simulink model "pyrolysis_adaptive_pid"  (R2024a)
settings: Solver=ode4  StartTime=0.0  StopTime=1800  FixedStep=0.05  RelTol=1e-3
InitFcn:
  | if ~exist('setpoint_ws','var'), setpoint_ws = 300; end
  | if ~exist('gs_enable_ws','var'), gs_enable_ws = 1; end
  | if ~exist('lambda_p_ws','var'), lambda_p_ws = 0.01; end
  | if ~exist('lambda_i_ws','var'), lambda_i_ws = 0.0001; end
  | if ~exist('lambda_d_ws','var'), lambda_d_ws = 0.003; end
  | if ~exist('noise_variance_ws','var'), noise_variance_ws = 2.25; end
undefined symbols (not defined in the file or in its folder): gs_enable_ws, lambda_d_ws, lambda_i_ws, lambda_p_ws, setpoint_ws
libraries: simulink x1
settings Model: Creator=indie  LastModifiedBy=indie

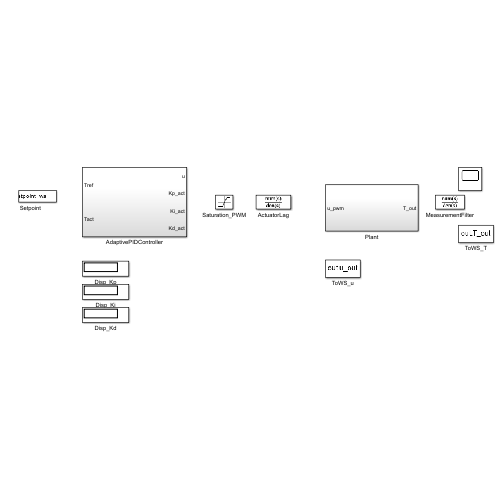
[thumbnail: Simulink's stored preview of the top-level diagram]
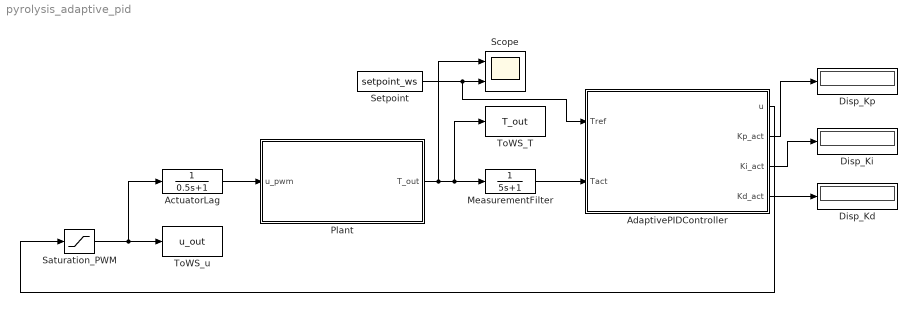
== system pyrolysis_adaptive_pid ==
  ActuatorLag : TransferFcn  Denominator=[0.5 1]
  AdaptivePIDController : Subsystem
  Disp_Kd : Display
  Disp_Ki : Display
  Disp_Kp : Display
  MeasurementFilter : TransferFcn  Denominator=[5 1]
  Plant : Subsystem
  Saturation_PWM : Saturate  UpperLimit=100  LowerLimit=0
  Scope : Scope  NumInputPorts=2
  Setpoint : Constant  Value=setpoint_ws
  ToWS_T : ToWorkspace  VariableName=T_out  SaveFormat=Timeseries  SampleTime=-1
  ToWS_u : ToWorkspace  VariableName=u_out  SaveFormat=Timeseries  SampleTime=-1
  wires:
  Saturation_PWM/1 -> ActuatorLag/1, ToWS_u/1
  ActuatorLag/1 -> Plant/1(u_pwm)
  Setpoint/1 -> Scope/2, AdaptivePIDController/1(Tref)
  MeasurementFilter/1 -> AdaptivePIDController/2(Tact)
  Plant/1(T_out) -> MeasurementFilter/1, ToWS_T/1, Scope/1
  AdaptivePIDController/3(Ki_act) -> Disp_Ki/1
  AdaptivePIDController/2(Kp_act) -> Disp_Kp/1
  AdaptivePIDController/1(u) -> Saturation_PWM/1
  AdaptivePIDController/4(Kd_act) -> Disp_Kd/1

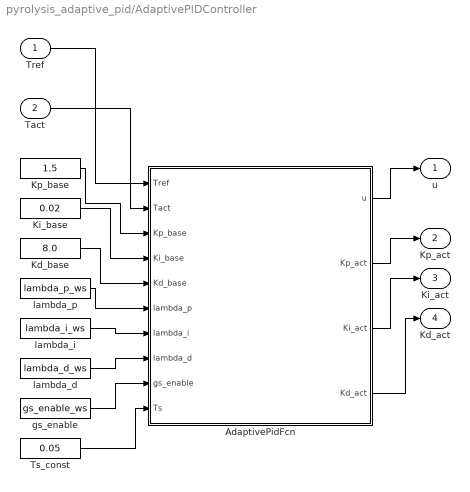
== system pyrolysis_adaptive_pid/AdaptivePIDController ==
  Tref : Inport
  Tact : Inport  Port=2
  AdaptivePidFcn : MATLAB Function  TreatAsAtomicUnit=on  SystemSampleTime=0.05
  Kd_base : Constant  Value=8.0
  Ki_base : Constant  Value=0.02
  Kp_base : Constant  Value=1.5
  Ts_const : Constant  Value=0.05
  gs_enable : Constant  Value=gs_enable_ws
  lambda_d : Constant  Value=lambda_d_ws
  lambda_i : Constant  Value=lambda_i_ws
  lambda_p : Constant  Value=lambda_p_ws
  u : Outport
  Kp_act : Outport  Port=2
  Ki_act : Outport  Port=3
  Kd_act : Outport  Port=4
  wires:
  ? -> ?
  Tref/1 -> AdaptivePidFcn/1(Tref)
  Tact/1 -> AdaptivePidFcn/2(Tact)
  Kp_base/1 -> AdaptivePidFcn/3(Kp_base)
  Ki_base/1 -> AdaptivePidFcn/4(Ki_base)
  Kd_base/1 -> AdaptivePidFcn/5(Kd_base)
  lambda_p/1 -> AdaptivePidFcn/6(lambda_p)
  lambda_i/1 -> AdaptivePidFcn/7(lambda_i)
  lambda_d/1 -> AdaptivePidFcn/8(lambda_d)
  gs_enable/1 -> AdaptivePidFcn/9(gs_enable)
  Ts_const/1 -> AdaptivePidFcn/10(Ts)
  AdaptivePidFcn/1(u) -> u/1
  AdaptivePidFcn/2(Kp_act) -> Kp_act/1
  AdaptivePidFcn/3(Ki_act) -> Ki_act/1
  AdaptivePidFcn/4(Kd_act) -> Kd_act/1

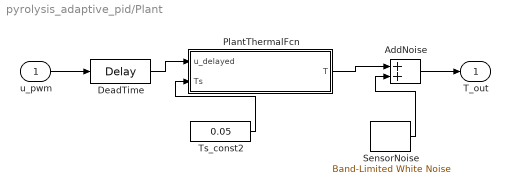
== system pyrolysis_adaptive_pid/Plant ==
  u_pwm : Inport
  AddNoise : Sum
  DeadTime : TransportDelay  DelayTime=15
  PlantThermalFcn : MATLAB Function  TreatAsAtomicUnit=on  SystemSampleTime=0.05
  SensorNoise : simulink/Sources/Band-Limited White Noise  Cov=noise_variance_ws  Ts=0.25  seed=23341
  Ts_const2 : Constant  Value=0.05
  T_out : Outport
  wires:
  ? -> ?
  u_pwm/1 -> DeadTime/1
  DeadTime/1 -> PlantThermalFcn/1(u_delayed)
  Ts_const2/1 -> PlantThermalFcn/2(Ts)
  PlantThermalFcn/1(T) -> AddNoise/1
  SensorNoise/1 -> AddNoise/2
  AddNoise/1 -> T_out/1

== matlab function pyrolysis_adaptive_pid/Plant/PlantThermalFcn ==
  data: u_delayed input; T output; Ts input
function T = plantThermalFcn(u_delayed, Ts)
%#codegen
% Model FOPDT nonlinear: gain K berubah per zona suhu, tau tetap.
% NILAI K, tau BERIKUT ADALAH ASUMSI/PLACEHOLDER -- kalibrasi ulang
% setelah tungku fisik diuji (belum ada data eksperimen nyata).
persistent T_state initialized
T_ambient = 30; K_base = 3.5; tau = 180;
if isempty(initialized)
    T_state = T_ambient;
    initialized = true;
end
T = T_state;
if T < 200
    Kz = K_base * 1.3;   % zona dingin
elseif T < 400
    Kz = K_base * 1.0;   % zona tengah (baseline)
else
    Kz = K_base * 0.7;   % zona panas
end
dT = (-(T_state - T_ambient) + Kz*u_delayed) / tau;
T_state = T_state + Ts*dT;
end

== matlab function pyrolysis_adaptive_pid/AdaptivePIDController/AdaptivePidFcn ==
  data: Tref input; u output; Tact input; Kp_base input; Ki_base input; Kd_base input; lambda_p input; lambda_i input; lambda_d input; gs_enable input; Ts input; Kp_act output; Ki_act output; Kd_act output
function [u, Kp_act, Ki_act, Kd_act] = adaptivePidFcn(Tref, Tact, Kp_base, Ki_base, Kd_base, lambda_p, lambda_i, lambda_d, gs_enable, Ts)
%#codegen
% Adaptive PID dua lapis:
%   Lapis 1 - gain scheduling per zona suhu (aktif bila gs_enable~=0)
%   Lapis 2 - adaptasi lambda (gain scheduling dinamis berbasis error),
%             dinonaktifkan (gains dibekukan di nilai dasar) selama
%             |e| <= DEAD_ZONE supaya tidak terus "berburu" di sekitar
%             setpoint akibat noise kecil (osilasi persisten).
persistent sum_e e_filt_prev initialized
if isempty(initialized)
    sum_e = 0; e_filt_prev = 0; initialized = true;
end

if gs_enable ~= 0
    if Tact < 200
        Kp = Kp_base*1.3; Ki = Ki_base*0.8; Kd = Kd_base*0.7;
    elseif Tact < 400
        Kp = Kp_base; Ki = Ki_base; Kd = Kd_base;
    else
        Kp = Kp_base*0.7; Ki = Ki_base*1.2; Kd = Kd_base*1.3;
    end
else
    Kp = Kp_base; Ki = Ki_base; Kd = Kd_base;
end

e = Tref - Tact;

% Derivative dari error yang DIFILTER (low-pass alpha=0.1), bukan
% error mentah -- meredam noise sensor supaya tidak memicu derivative
% kick / lonjakan adaptasi lambda tiap sample.
alpha = 0.1;
e_filt = alpha*e + (1-alpha)*e_filt_prev;
delta_e = (e_filt - e_filt_prev) / Ts;
e_filt_prev = e_filt;

% Coba akumulasi integral (trial) -- baru dikonfirmasi/dibatalkan
% oleh logika anti-windup di bawah.
sum_e_trial = sum_e + e*Ts;

DEAD_ZONE = 8.0; % degC
if abs(e) > DEAD_ZONE
    Kp_act = Kp + lambda_p*abs(e);
    Ki_act = Ki + lambda_i*abs(sum_e_trial);
    Kd_act = Kd + lambda_d*abs(delta_e);
else
    % Dekat setpoint: bekukan gain di nilai dasar, jangan adapt.
    Kp_act = Kp;
    Ki_act = Ki;
    Kd_act = Kd;
end

u_trial = Kp_act*e + Ki_act*sum_e_trial + Kd_act*delta_e;
u = min(max(u_trial, 0), 100);

% Anti-windup: integrator HANYA diperbarui jika output TIDAK saturasi.
% Tanpa ini, saat pemanasan panjang dari 30 degC ke setpoint (mis. 300
% degC), error besar terus menumpuk di sum_e ("integrator windup")
% walau keluaran sudah mentok 100%; begitu suhu mendekati setpoint,
% sum_e yang sudah "menggunung" itu membuat u tetap besar terlalu
% lama, menyebabkan overshoot parah.
if u_trial == u
    sum_e = sum_e_trial;
elseif abs(e) > DEAD_ZONE
    Ki_act = Ki + lambda_i*abs(sum_e); % integrator dibekukan, tampilkan nilai lama
end
end
